simulink model "videoOutput"  (R2016a)
settings: Solver=FixedStepDiscrete  StartTime=0.0  StopTime=inf  FixedStep=.1  RelTol=1e-3
libraries: visionsinks x2, LibrarySimulinkSAS x2, sldrtlib x1
settings Model: Creator=DSANTIAGO  LastModifiedBy=DSANTIAGO

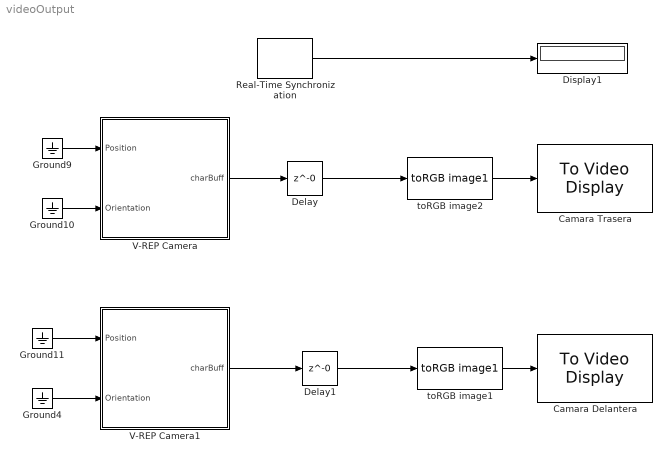
== system videoOutput ==
  Camara Delantera : visionsinks/To Video Display  windowSizeMode=Normal  openAtMdlStart=on  fullScreen=off  videoWindowX=0  videoWindowY=22  saveWindowSize=off  videoWindowWidth=1360  videoWindowHeight=706  inputColorFormat=RGB  inputType=Obsolete  imagePorts=One multidimensional signal  OutputDevice=On-screen video monitor  dataOrg=Column-major  isWindowOpen=off
  Camara Trasera : visionsinks/To Video Display  windowSizeMode=Normal  openAtMdlStart=on  fullScreen=off  videoWindowX=1360  videoWindowY=22  saveWindowSize=off  videoWindowWidth=1360  videoWindowHeight=746  inputColorFormat=RGB  inputType=Obsolete  imagePorts=One multidimensional signal  OutputDevice=On-screen video monitor  dataOrg=Column-major  isWindowOpen=off
  Delay : Delay  DelayLength=0
  Delay1 : Delay  DelayLength=0
  Display1 : Display
  Ground{4,9..11} (4 alike) : Ground
  Real-Time Synchronization : sldrtlib/Real-Time Synchronization  SampleTime=0.1  MaxMissedTicks=inf  ShowMissedTicks=on  YieldWhenWaiting=off
  V-REP Camera : Subsystem  mask{ResX=256, ResY=128, id=4}
      mask prompts: ResX "Resolucion Camara X"; ResY "Resolucion Camara Y"; id "Id Memoria Compartida"
      mask Display:
      | image('webcam.jpg')
      | color('red');
      | port_label('input',1,'Posicion')
      | port_label('input',2,'Orientacion')
      | port_label('output',1,'Char Buffer')
  V-REP Camera1 : Subsystem  mask{ResX=256, ResY=128, id=16}
      mask prompts: ResX "Resolucion Camara X"; ResY "Resolucion Camara Y"; id "Id Memoria Compartida"
      mask Display:
      | image('webcam.jpg')
      | color('red');
      | port_label('input',1,'Posicion')
      | port_label('input',2,'Orientacion')
      | port_label('output',1,'Char Buffer')
  toRGB image1 : LibrarySimulinkSAS/V-REP Camera/toRGB image1  ResX=256  ResY=128
  toRGB image2 : LibrarySimulinkSAS/V-REP Camera/toRGB image1  ResX=256  ResY=128
  wires:
  Ground9/1 -> V-REP Camera/1("Position ")
  Ground10/1 -> V-REP Camera/2(Orientation)
  Delay/1 -> toRGB image2/1
  V-REP Camera/1(charBuff) -> Delay/1
  toRGB image2/1 -> Camara Trasera/1
  Ground11/1 -> V-REP Camera1/1("Position ")
  Ground4/1 -> V-REP Camera1/2(Orientation)
  Delay1/1 -> toRGB image1/1
  V-REP Camera1/1(charBuff) -> Delay1/1
  toRGB image1/1 -> Camara Delantera/1
  Real-Time Synchronization/1 -> Display1/1

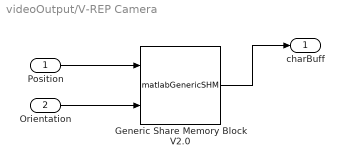
== system videoOutput/V-REP Camera ==
  "Position " : Inport
  Orientation : Inport  Port=2
  Generic Share Memory Block V2.0 : S-Function  FunctionName=matlabGenericSHM  Parameters=nombre,dispositivo,vecE,vecS,tipoE,tipoS  SFunctionDeploymentMode=off  EnableBusSupport=off  mask(Generic Share Memory block V2.0){nombre='vrepCam', dispositivo=id, vecE=[3 3], vecS=[3*ResX*ResY], tipoE=['f' 'f'], tipoS=['C']}
      mask prompts: nombre "Share Memory base name"; dispositivo "Device Number"; vecE "Sizes input vector"; vecS "Sizes output vector"; tipoE "Data Types Inputs"; tipoS "Data Types Outputs"
      mask help:
      | This block allows Simulink communication with external processes through shared memory. It works on Unix and Windows.
      | More information in Help.
      mask Help:
      | Share Memory base name (nombre): It's the base string of share memory ej 'robot'
      | Device Number (dispositivo): integer that identifies the device between multiple in use
      | Two shared memorys are created with names:
      | "%name_entrada_%dispositivo" for the device input (writing)
      | "%name_salida_%dispositivo" for the device output (reading)
      | Sizes input vector (vecE)  : array that specify the number of inputs (array dimension) and the inputs size (array values)
      | Sizes output vector  (vecS): array that specify the number of outputs (array dimension) and the outputs size (array values)
      | Data types input(tipoE): char array that specify each input types
      | Data types output (tipoS): char array that specify each output types
      | Allowed types are:
      | ('f'=float, 'd'=double, 'i'=int32, 'c'=char, 'C'= unsigned char, 'I'=unsigned int)
      | Example.
      | Suppose the following parameters:
      | nombre='exampleMemory'
      | dispositivo=10
      | vecE=[3 2 1]
      | vecS=[6 5 7 8]
      | tipoE=['f' 'I' 'c']
      | tipoS=['C' 'i' 'd' 'd']
      | 
      | Two Share Memories are created with names:
      | "exampleMemory_entrada_10" (block input)
      | "exampleMemory_salida_10"  (block output)
      | 3 inputs are created:
      |  1° Dimension 3, type "unsigned char"
      |  2° Dimension 2, type "int"
      |  3° Dimension 1, type "char"
      | 4 outputs are created:
      |  1° Dimension 6, type "float"
      |  2° Dimension 5, type "unsigned int"
      |  3° Dimension 7, type "double"
      |  3° Dimension 8, type "double"
      mask Display: image('shmem.jpg')
  charBuff : Outport
  wires:
  Generic Share Memory Block V2.0/1 -> charBuff/1
  Orientation/1 -> Generic Share Memory Block V2.0/2
  "Position "/1 -> Generic Share Memory Block V2.0/1

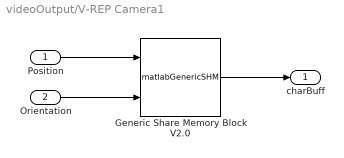
== system videoOutput/V-REP Camera1 ==
  "Position " : Inport
  Orientation : Inport  Port=2
  Generic Share Memory Block V2.0 : S-Function  FunctionName=matlabGenericSHM  Parameters=nombre,dispositivo,vecE,vecS,tipoE,tipoS  SFunctionDeploymentMode=off  EnableBusSupport=off  mask(Generic Share Memory block V2.0){nombre='vrepCam', dispositivo=id, vecE=[3 3], vecS=[3*ResX*ResY], tipoE=['f' 'f'], tipoS=['C']}
      mask prompts: nombre "Share Memory base name"; dispositivo "Device Number"; vecE "Sizes input vector"; vecS "Sizes output vector"; tipoE "Data Types Inputs"; tipoS "Data Types Outputs"
      mask help:
      | This block allows Simulink communication with external processes through shared memory. It works on Unix and Windows.
      | More information in Help.
      mask Help:
      | Share Memory base name (nombre): It's the base string of share memory ej 'robot'
      | Device Number (dispositivo): integer that identifies the device between multiple in use
      | Two shared memorys are created with names:
      | "%name_entrada_%dispositivo" for the device input (writing)
      | "%name_salida_%dispositivo" for the device output (reading)
      | Sizes input vector (vecE)  : array that specify the number of inputs (array dimension) and the inputs size (array values)
      | Sizes output vector  (vecS): array that specify the number of outputs (array dimension) and the outputs size (array values)
      | Data types input(tipoE): char array that specify each input types
      | Data types output (tipoS): char array that specify each output types
      | Allowed types are:
      | ('f'=float, 'd'=double, 'i'=int32, 'c'=char, 'C'= unsigned char, 'I'=unsigned int)
      | Example.
      | Suppose the following parameters:
      | nombre='exampleMemory'
      | dispositivo=10
      | vecE=[3 2 1]
      | vecS=[6 5 7 8]
      | tipoE=['f' 'I' 'c']
      | tipoS=['C' 'i' 'd' 'd']
      | 
      | Two Share Memories are created with names:
      | "exampleMemory_entrada_10" (block input)
      | "exampleMemory_salida_10"  (block output)
      | 3 inputs are created:
      |  1° Dimension 3, type "unsigned char"
      |  2° Dimension 2, type "int"
      |  3° Dimension 1, type "char"
      | 4 outputs are created:
      |  1° Dimension 6, type "float"
      |  2° Dimension 5, type "unsigned int"
      |  3° Dimension 7, type "double"
      |  3° Dimension 8, type "double"
      mask Display: image('shmem.jpg')
  charBuff : Outport
  wires:
  Generic Share Memory Block V2.0/1 -> charBuff/1
  Orientation/1 -> Generic Share Memory Block V2.0/2
  "Position "/1 -> Generic Share Memory Block V2.0/1
